simulink model "CrusieControl"  (R2020b)
settings: Solver=VariableStepAuto  StartTime=0.0  StopTime=120  RelTol=1e-3
model workspace (MAT data in the model file):
  Kd = Simulink.Parameter
  Kd.Value = 40
  Kd.DataType = 'auto'
  Kd.Dimensions = [1 1]
  Ki = Simulink.Parameter
  Ki.Value = 40
  Ki.DataType = 'auto'
  Ki.Dimensions = [1 1]
  Kp = Simulink.Parameter
  Kp.Value = 800
  Kp.DataType = 'auto'
  Kp.Dimensions = [1 1]
settings Model: Creator=gokul  LastModifiedBy=gokul
settings DataIOCC: SaveOutput=off  SaveTime=off

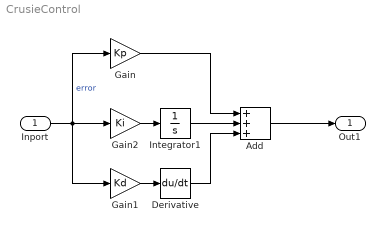
== system CrusieControl ==
  Inport : Inport  OutDataTypeStr=double  PortDimensions=1  SampleTime=0
  Add : Sum  Inputs=+++
  Derivative : Derivative
  Gain : Gain  Gain=Kp
  Gain1 : Gain  Gain=Kd
  Gain2 : Gain  Gain=Ki
  Integrator1 : Integrator
  Out1 : Outport  OutDataTypeStr=double  PortDimensions=1  SampleTime=0
  wires:
  Gain/1 -> Add/1
  Derivative/1 -> Add/3
  Inport/1 -> Gain1/1, Gain/1, Gain2/1  "error"
  Gain1/1 -> Derivative/1
  Integrator1/1 -> Add/2
  Add/1 -> Out1/1
  Gain2/1 -> Integrator1/1
